simulink model "dynamicsubsystems"  (R2018a)
settings: Solver=VariableStepAuto  StartTime=0.0  StopTime=10.0  RelTol=1e-3
settings Model: Creator=kartik  LastModifiedBy=kartik

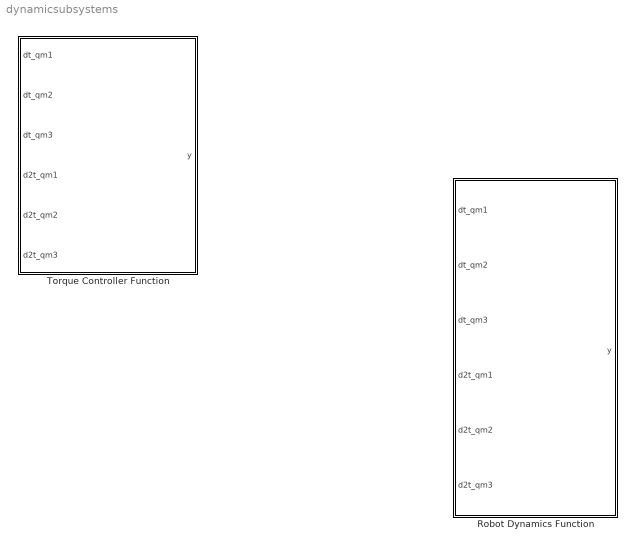
== system dynamicsubsystems ==
  Robot Dynamics Function : MATLAB Function  TreatAsAtomicUnit=on
  Torque Controller Function : MATLAB Function  TreatAsAtomicUnit=on

== matlab function dynamicsubsystems/Robot Dynamics Function ==
  data: y output; dt_qm1 input; dt_qm2 input; dt_qm3 input; d2t_qm1 input; d2t_qm2 input; d2t_qm3 input
function y = OmniRobotDynamics(dt_qm1, dt_qm2, dt_qm3, d2t_qm1, d2t_qm2, d2t_qm3)

% Define Constants
Jm = 2.7e-07;
Jl = 8e-5;
J = 4.6e-3;
r = 0.02;
L = 0.07;
n = 14;
m = 2.36;
Cm = 5e-8;
Cl = 0;


% Define Dynamic Parameters
k1 = Jm + (Jl/(n.^2)) + ((r.^2)/(n.^2))*(0.2810*m + 11.75*J);
k2 = ((r.^2)/(n.^2))*(0.03812*m + 11.75*J);
k3 = ((r.^2)/(n.^2))*(-0.2619*m + 9.050*J);
k4 = ((r.^2)/(n.^2))*(-0.05717*m + 9.050*J);
k5 = Jm + (Jl/(n.^2)) + ((r.^2)/(n.^2))*(0.2459*m + 6.9710*J);
k6 = ((r.^2)/(n.^2))*(0.07323*m + 6.9710*J);
k7 = Cm + (Cl/(n.^2));
k8 = 0.2784*(r.^2)/(n.^2)*m;
k9 = 0.02184*(r.^2)/(n.^2)*m;
k10 = 0.2566*(r.^2)/(n.^2)*m;
k11 = 0.2347*(r.^2)/(n.^2)*m;

dt_phi = r*(dt_qm1 + dt_qm2 + dt_qm3)/(2*n*L);
dt_qm = [dt_qm1 dt_qm2 dt_qm3];
d2t_qm = [d2t_qm1 d2t_qm2 d2t_qm3];

% Define Dynamic Parametric Matrices
Z = [k1 k2 k3 k4;
     k2 k1 k4 k3;
     k3 k4 k5 k6;
     k4 k3 k6 k5];

V = [k7 -k8*dt_phi k9*dt_phi k10*dt_phi;
     k8*dt_phi k7 -k10*dt_phi -k9*dt_phi;
     -k9*dt_phi k10*dt_phi k7 -k11*dt_phi;
     -k10*dt_phi k9*dt_phi k11*dt_phi k7];

Tm = Z*d2t_qm' + V*dt_qm';
y = Tm;

== matlab function dynamicsubsystems/Torque Controller Function ==
  data: dt_qm1 input; y output; dt_qm2 input; dt_qm3 input; d2t_qm1 input; d2t_qm2 input; d2t_qm3 input
function y = TorqueDynamics(dt_qm1, dt_qm2, dt_qm3, d2t_qm1, d2t_qm2, d2t_qm3)

% Define Constants
Jm = 2.7e-07;
Jl = 8e-5;
J = 4.6e-3;
r = 0.02;
n = 14;
m = 2.36;
Cm = 5e-8;
Cl = 0;

% Define Dynamic Parameters
k1 = Jm + (Jl/(n.^2)) + (((4*m*(L.^2) + J)*r.^2)/(9*L.^2*n.^2));
k2 = (((-2*m*(L.^2) + J)*r.^2)/(9*L.^2*n.^2));
k3 = Cm + (Cl/(n.^2));
k4 = (3.4641*m*r.^2)/(9*n.^2);
klr = 1/8.71;
km = 0.0144;
ke = 0.0145;

dt_phi = r*(dt_qm1 + dt_qm2 + dt_qm3)/(2*n*L);
dt_qm = [dt_qm1 dt_qm2 dt_qm3];
d2t_qm = [d2t_qm1 d2t_qm2 d2t_qm3];

% Coupled nonlinear equations of motion at actuator level
E = (k1/(klr*km))*[1 0 0; 0 1 0; 0 0 1]*d2t_qm' +... 
    (k2/(klr*km))*[0 1 1; 1 0 1; 1 1 0]*d2t_qm' + ...
    ((k3/klr*km) +ke)*[1 0 0; 0 1 0; 0 0 1]*dt_qm' + ...
    ((k4*dt_phi)/(klr*km))*[0 1 -1; -1 0 1; 1 -1 0]*dt_qm';

% Eqns pertaining to Torque Dynamics
Tm = (E - ke*(dt_qm'))*klr*km;
y = Tm;
